simulink model "TST_AirCtl_Mon"  (R2016b)
settings: Solver=FixedStepDiscrete  StartTime=0.0  StopTime=simTime  FixedStep=sampleTime  RelTol=1e-3
values from neighbouring files (symbols this model uses):
  testCase = 1    [initTST_AirCtl_Mon_001.m]
libraries: simulink x8, UnitTest_Lib x6
settings Model: Creator=zhulinfeng  LastModifiedBy=zhulinfeng
settings DebuggingCC: SignalRangeChecking=error

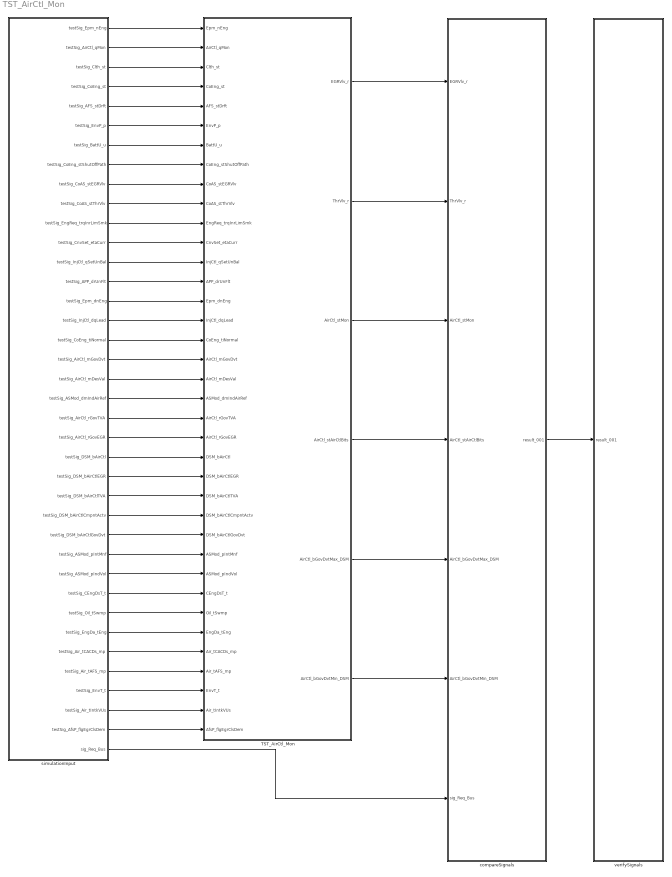
== system TST_AirCtl_Mon ==
  TST_AirCtl_Mon : Subsystem
  compareSignals : Subsystem
  simulationInput : Subsystem
  verifySignals : Subsystem
  wires:
  simulationInput/1(testSig_Epm_nEng) -> TST_AirCtl_Mon/1(Epm_nEng)
  simulationInput/2(testSig_AirCtl_qMon) -> TST_AirCtl_Mon/2(AirCtl_qMon)
  simulationInput/3(testSig_Clth_st) -> TST_AirCtl_Mon/3(Clth_st)
  simulationInput/4(testSig_CoEng_st) -> TST_AirCtl_Mon/4(CoEng_st)
  simulationInput/5(testSig_AFS_stDrft) -> TST_AirCtl_Mon/5(AFS_stDrft)
  simulationInput/6(testSig_EnvP_p) -> TST_AirCtl_Mon/6(EnvP_p)
  simulationInput/7(testSig_BattU_u) -> TST_AirCtl_Mon/7(BattU_u)
  simulationInput/8(testSig_CoEng_stShutOffPath) -> TST_AirCtl_Mon/8(CoEng_stShutOffPath)
  simulationInput/9(testSig_CoAS_stEGRVlv) -> TST_AirCtl_Mon/9(CoAS_stEGRVlv)
  simulationInput/10(testSig_CoAS_stThrVlv) -> TST_AirCtl_Mon/10(CoAS_stThrVlv)
  simulationInput/11(testSig_EngReq_trqInrLimSmk) -> TST_AirCtl_Mon/11(EngReq_trqInrLimSmk)
  simulationInput/12(testSig_CnvSet_etaCurr) -> TST_AirCtl_Mon/12(CnvSet_etaCurr)
  simulationInput/13(testSig_InjCtl_qSetUnBal) -> TST_AirCtl_Mon/13(InjCtl_qSetUnBal)
  simulationInput/14(testSig_APP_drUnFlt) -> TST_AirCtl_Mon/14(APP_drUnFlt)
  simulationInput/15(testSig_Epm_dnEng) -> TST_AirCtl_Mon/15(Epm_dnEng)
  simulationInput/16(testSig_InjCtl_dqLead) -> TST_AirCtl_Mon/16(InjCtl_dqLead)
  simulationInput/17(testSig_CoEng_tiNormal) -> TST_AirCtl_Mon/17(CoEng_tiNormal)
  simulationInput/18(testSig_AirCtl_mGovDvt) -> TST_AirCtl_Mon/18(AirCtl_mGovDvt)
  simulationInput/19(testSig_AirCtl_mDesVal) -> TST_AirCtl_Mon/19(AirCtl_mDesVal)
  simulationInput/20(testSig_ASMod_dmIndAirRef) -> TST_AirCtl_Mon/20(ASMod_dmIndAirRef)
  simulationInput/21(testSig_AirCtl_rGovTVA) -> TST_AirCtl_Mon/21(AirCtl_rGovTVA)
  simulationInput/22(testSig_AirCtl_rGovEGR) -> TST_AirCtl_Mon/22(AirCtl_rGovEGR)
  simulationInput/23(testSig_DSM_bAirCtl) -> TST_AirCtl_Mon/23(DSM_bAirCtl)
  simulationInput/24(testSig_DSM_bAirCtlEGR) -> TST_AirCtl_Mon/24(DSM_bAirCtlEGR)
  simulationInput/25(testSig_DSM_bAirCtlTVA) -> TST_AirCtl_Mon/25(DSM_bAirCtlTVA)
  simulationInput/26(testSig_DSM_bAirCtlCmpntActv) -> TST_AirCtl_Mon/26(DSM_bAirCtlCmpntActv)
  simulationInput/27(testSig_DSM_bAirCtlGovDvt) -> TST_AirCtl_Mon/27(DSM_bAirCtlGovDvt)
  simulationInput/28(testSig_ASMod_pIntMnf) -> TST_AirCtl_Mon/28(ASMod_pIntMnf)
  simulationInput/29(testSig_ASMod_pIndVol) -> TST_AirCtl_Mon/29(ASMod_pIndVol)
  simulationInput/30(testSig_CEngDsT_t) -> TST_AirCtl_Mon/30(CEngDsT_t)
  simulationInput/31(testSig_Oil_tSwmp) -> TST_AirCtl_Mon/31(Oil_tSwmp)
  simulationInput/32(testSig_EngDa_tEng) -> TST_AirCtl_Mon/32(EngDa_tEng)
  simulationInput/33(testSig_Air_tCACDs_mp) -> TST_AirCtl_Mon/33(Air_tCACDs_mp)
  simulationInput/34(testSig_Air_tAFS_mp) -> TST_AirCtl_Mon/34(Air_tAFS_mp)
  simulationInput/35(testSig_EnvT_t) -> TST_AirCtl_Mon/35(EnvT_t)
  simulationInput/36(testSig_Air_tIntkVUs) -> TST_AirCtl_Mon/36(Air_tIntkVUs)
  simulationInput/37(testSig_AfsP_flgEgrClsDem) -> TST_AirCtl_Mon/37(AfsP_flgEgrClsDem)
  TST_AirCtl_Mon/1(EGRVlv_r) -> compareSignals/1(EGRVlv_r)
  TST_AirCtl_Mon/2(ThrVlv_r) -> compareSignals/2(ThrVlv_r)
  TST_AirCtl_Mon/3(AirCtl_stMon) -> compareSignals/3(AirCtl_stMon)
  TST_AirCtl_Mon/4(AirCtl_stAirCtlBits) -> compareSignals/4(AirCtl_stAirCtlBits)
  TST_AirCtl_Mon/5(AirCtl_bGovDvtMax_DSM) -> compareSignals/5(AirCtl_bGovDvtMax_DSM)
  TST_AirCtl_Mon/6(AirCtl_bGovDvtMin_DSM) -> compareSignals/6(AirCtl_bGovDvtMin_DSM)
  simulationInput/38(sig_Req_Bus) -> compareSignals/7(sig_Req_Bus)
  compareSignals/1(result_001) -> verifySignals/1(result_001)

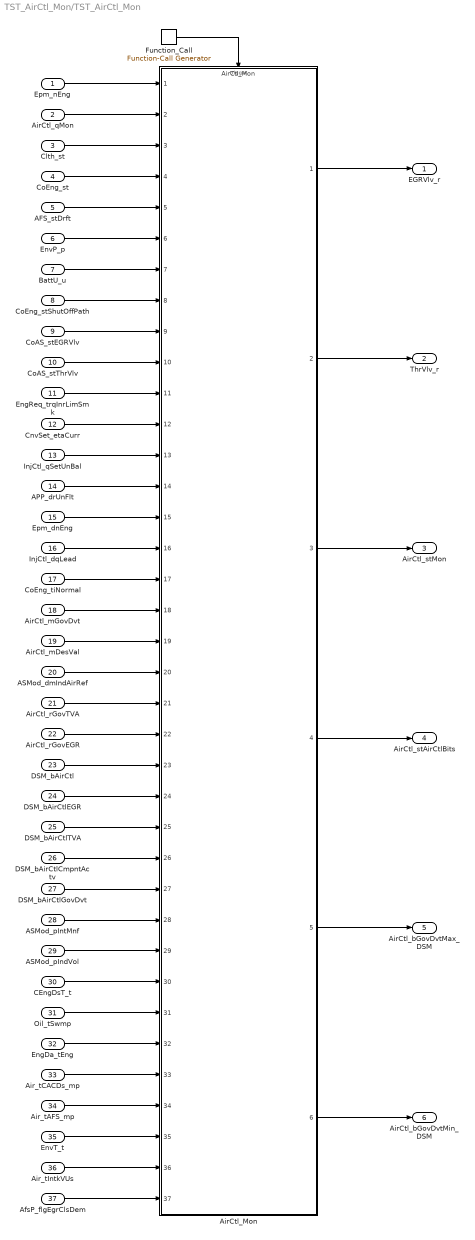
== system TST_AirCtl_Mon/TST_AirCtl_Mon ==
  Epm_nEng : Inport
  AirCtl_qMon : Inport  Port=2
  Clth_st : Inport  Port=3
  CoEng_st : Inport  Port=4
  AFS_stDrft : Inport  Port=5
  EnvP_p : Inport  Port=6
  BattU_u : Inport  Port=7
  CoEng_stShutOffPath : Inport  Port=8
  CoAS_stEGRVlv : Inport  Port=9
  CoAS_stThrVlv : Inport  Port=10
  EngReq_trqInrLimSmk : Inport  Port=11
  CnvSet_etaCurr : Inport  Port=12
  InjCtl_qSetUnBal : Inport  Port=13
  APP_drUnFlt : Inport  Port=14
  Epm_dnEng : Inport  Port=15
  InjCtl_dqLead : Inport  Port=16
  CoEng_tiNormal : Inport  Port=17
  AirCtl_mGovDvt : Inport  Port=18
  AirCtl_mDesVal : Inport  Port=19
  ASMod_dmIndAirRef : Inport  Port=20
  AirCtl_rGovTVA : Inport  Port=21
  AirCtl_rGovEGR : Inport  Port=22
  DSM_bAirCtl : Inport  Port=23
  DSM_bAirCtlEGR : Inport  Port=24
  DSM_bAirCtlTVA : Inport  Port=25
  DSM_bAirCtlCmpntActv : Inport  Port=26
  DSM_bAirCtlGovDvt : Inport  Port=27
  ASMod_pIntMnf : Inport  Port=28
  ASMod_pIndVol : Inport  Port=29
  CEngDsT_t : Inport  Port=30
  Oil_tSwmp : Inport  Port=31
  EngDa_tEng : Inport  Port=32
  Air_tCACDs_mp : Inport  Port=33
  Air_tAFS_mp : Inport  Port=34
  EnvT_t : Inport  Port=35
  Air_tIntkVUs : Inport  Port=36
  AfsP_flgEgrClsDem : Inport  Port=37
  AirCtl_Mon : ModelReference  ModelNameDialog=AirCtl_Mon  SimulationMode=Normal  ModelReferenceVersion=1.83  TriggerPortName=function  TriggerPortTriggerType=function-call  TriggerPortStatesWhenEnabling=held
  Function_Call : simulink/Ports & Subsystems/Function-Call Generator  sample_time=sampleTime  numberOfIterations=1
  EGRVlv_r : Outport
  ThrVlv_r : Outport  Port=2
  AirCtl_stMon : Outport  Port=3
  AirCtl_stAirCtlBits : Outport  Port=4
  AirCtl_bGovDvtMax_DSM : Outport  Port=5
  AirCtl_bGovDvtMin_DSM : Outport  Port=6
  wires:
  Function_Call/1 -> AirCtl_Mon/Trigger
  Epm_nEng/1 -> AirCtl_Mon/1
  AirCtl_qMon/1 -> AirCtl_Mon/2
  Clth_st/1 -> AirCtl_Mon/3
  CoEng_st/1 -> AirCtl_Mon/4
  AFS_stDrft/1 -> AirCtl_Mon/5
  EnvP_p/1 -> AirCtl_Mon/6
  BattU_u/1 -> AirCtl_Mon/7
  CoEng_stShutOffPath/1 -> AirCtl_Mon/8
  CoAS_stEGRVlv/1 -> AirCtl_Mon/9
  CoAS_stThrVlv/1 -> AirCtl_Mon/10
  EngReq_trqInrLimSmk/1 -> AirCtl_Mon/11
  CnvSet_etaCurr/1 -> AirCtl_Mon/12
  InjCtl_qSetUnBal/1 -> AirCtl_Mon/13
  APP_drUnFlt/1 -> AirCtl_Mon/14
  Epm_dnEng/1 -> AirCtl_Mon/15
  InjCtl_dqLead/1 -> AirCtl_Mon/16
  CoEng_tiNormal/1 -> AirCtl_Mon/17
  AirCtl_mGovDvt/1 -> AirCtl_Mon/18
  AirCtl_mDesVal/1 -> AirCtl_Mon/19
  ASMod_dmIndAirRef/1 -> AirCtl_Mon/20
  AirCtl_rGovTVA/1 -> AirCtl_Mon/21
  AirCtl_rGovEGR/1 -> AirCtl_Mon/22
  DSM_bAirCtl/1 -> AirCtl_Mon/23
  DSM_bAirCtlEGR/1 -> AirCtl_Mon/24
  DSM_bAirCtlTVA/1 -> AirCtl_Mon/25
  DSM_bAirCtlCmpntActv/1 -> AirCtl_Mon/26
  DSM_bAirCtlGovDvt/1 -> AirCtl_Mon/27
  ASMod_pIntMnf/1 -> AirCtl_Mon/28
  ASMod_pIndVol/1 -> AirCtl_Mon/29
  CEngDsT_t/1 -> AirCtl_Mon/30
  Oil_tSwmp/1 -> AirCtl_Mon/31
  EngDa_tEng/1 -> AirCtl_Mon/32
  Air_tCACDs_mp/1 -> AirCtl_Mon/33
  Air_tAFS_mp/1 -> AirCtl_Mon/34
  EnvT_t/1 -> AirCtl_Mon/35
  Air_tIntkVUs/1 -> AirCtl_Mon/36
  AfsP_flgEgrClsDem/1 -> AirCtl_Mon/37
  AirCtl_Mon/1 -> EGRVlv_r/1
  AirCtl_Mon/2 -> ThrVlv_r/1
  AirCtl_Mon/3 -> AirCtl_stMon/1
  AirCtl_Mon/4 -> AirCtl_stAirCtlBits/1
  AirCtl_Mon/5 -> AirCtl_bGovDvtMax_DSM/1
  AirCtl_Mon/6 -> AirCtl_bGovDvtMin_DSM/1

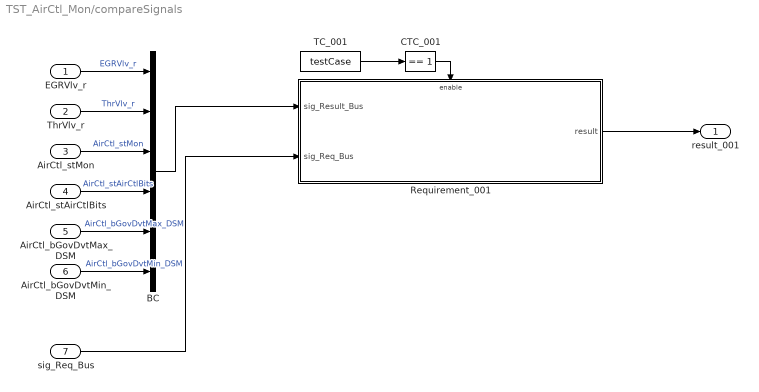
== system TST_AirCtl_Mon/compareSignals ==
  EGRVlv_r : Inport
  ThrVlv_r : Inport  Port=2
  AirCtl_stMon : Inport  Port=3
  AirCtl_stAirCtlBits : Inport  Port=4
  AirCtl_bGovDvtMax_DSM : Inport  Port=5
  AirCtl_bGovDvtMin_DSM : Inport  Port=6
  sig_Req_Bus : Inport  Port=7
  BC : BusCreator  Inputs=6
  CTC_001 : simulink/Logic and Bit Operations/Compare To Constant  relop===  const=1  OutDataTypeStr=boolean
  Requirement_001 : Subsystem
  TC_001 : Constant  Value=testCase
  result_001 : Outport
  wires:
  EGRVlv_r/1 -> BC/1  "EGRVlv_r"
  ThrVlv_r/1 -> BC/2  "ThrVlv_r"
  AirCtl_stMon/1 -> BC/3  "AirCtl_stMon"
  AirCtl_stAirCtlBits/1 -> BC/4  "AirCtl_stAirCtlBits"
  AirCtl_bGovDvtMax_DSM/1 -> BC/5  "AirCtl_bGovDvtMax_DSM"
  AirCtl_bGovDvtMin_DSM/1 -> BC/6  "AirCtl_bGovDvtMin_DSM"
  TC_001/1 -> CTC_001/1
  CTC_001/1 -> Requirement_001/Enable
  sig_Req_Bus/1 -> Requirement_001/2(sig_Req_Bus)
  BC/1 -> Requirement_001/1(sig_Result_Bus)
  Requirement_001/1(result) -> result_001/1

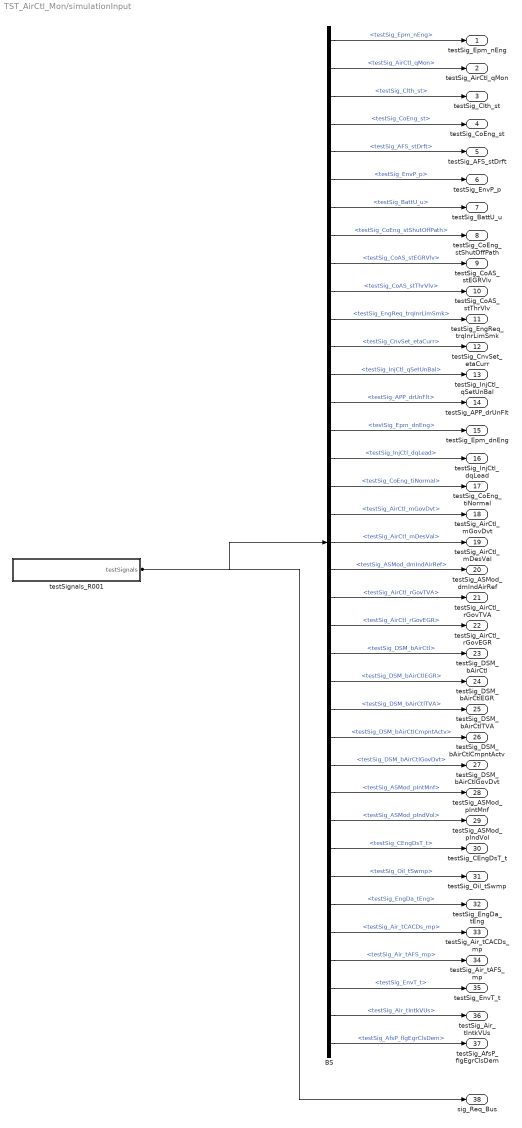
== system TST_AirCtl_Mon/simulationInput ==
  BS : BusSelector  OutputSignals=testSig_Epm_nEng,testSig_AirCtl_qMon,testSig_Clth_st,testSig_CoEng_st,testSig_AFS_stDrft,testSig_EnvP_p,testSig_BattU_u,testSig_CoEng_stShutOffPath,testSig_CoAS_stEGRVlv,testSig_CoAS_stThrVlv,testSig_EngReq_trqInrLimSmk,testSig_CnvSet_etaCurr,testSig_InjCtl_qSetUnBal,testSig_APP_drUnFlt,testSig_Epm_dnEng,testSig_InjCtl_dqLead,testSig_CoEng_tiNormal,testSig_AirCtl_mGovDvt,testSig_AirCtl_mDesVal,testSig_ASMod_dmIndAirRef,testSig_AirCtl_rGovTVA,testSig_AirCtl_rGovEGR,testSig_DSM_bAirCtl,testSig_DSM_bAirCtlEGR,testSig_DSM_bAirCtlTVA,testSig_DSM_bAirCtlCmpntActv,testSig_DSM_bAirCtlGovDvt,testSig_ASMod_pIntMnf,testSig_ASMod_pIndVol,testSig_CEngDsT_t,testSig_Oil_tSwmp,testSig_EngDa_tEng,testSig_Air_tCACDs_mp,testSig_Air_tAFS_mp,testSig_EnvT_t,testSig_Air_tIntkVUs,testSig_AfsP_flgEgrClsDem
  testSignals_R001 : Subsystem
  testSig_Epm_nEng : Outport
  testSig_AirCtl_qMon : Outport  Port=2
  testSig_Clth_st : Outport  Port=3
  testSig_CoEng_st : Outport  Port=4
  testSig_AFS_stDrft : Outport  Port=5
  testSig_EnvP_p : Outport  Port=6
  testSig_BattU_u : Outport  Port=7
  testSig_CoEng_stShutOffPath : Outport  Port=8
  testSig_CoAS_stEGRVlv : Outport  Port=9
  testSig_CoAS_stThrVlv : Outport  Port=10
  testSig_EngReq_trqInrLimSmk : Outport  Port=11
  testSig_CnvSet_etaCurr : Outport  Port=12
  testSig_InjCtl_qSetUnBal : Outport  Port=13
  testSig_APP_drUnFlt : Outport  Port=14
  testSig_Epm_dnEng : Outport  Port=15
  testSig_InjCtl_dqLead : Outport  Port=16
  testSig_CoEng_tiNormal : Outport  Port=17
  testSig_AirCtl_mGovDvt : Outport  Port=18
  testSig_AirCtl_mDesVal : Outport  Port=19
  testSig_ASMod_dmIndAirRef : Outport  Port=20
  testSig_AirCtl_rGovTVA : Outport  Port=21
  testSig_AirCtl_rGovEGR : Outport  Port=22
  testSig_DSM_bAirCtl : Outport  Port=23
  testSig_DSM_bAirCtlEGR : Outport  Port=24
  testSig_DSM_bAirCtlTVA : Outport  Port=25
  testSig_DSM_bAirCtlCmpntActv : Outport  Port=26
  testSig_DSM_bAirCtlGovDvt : Outport  Port=27
  testSig_ASMod_pIntMnf : Outport  Port=28
  testSig_ASMod_pIndVol : Outport  Port=29
  testSig_CEngDsT_t : Outport  Port=30
  testSig_Oil_tSwmp : Outport  Port=31
  testSig_EngDa_tEng : Outport  Port=32
  testSig_Air_tCACDs_mp : Outport  Port=33
  testSig_Air_tAFS_mp : Outport  Port=34
  testSig_EnvT_t : Outport  Port=35
  testSig_Air_tIntkVUs : Outport  Port=36
  testSig_AfsP_flgEgrClsDem : Outport  Port=37
  sig_Req_Bus : Outport  Port=38
  wires:
  BS/1 -> testSig_Epm_nEng/1  "<testSig_Epm_nEng>"
  BS/2 -> testSig_AirCtl_qMon/1  "<testSig_AirCtl_qMon>"
  BS/3 -> testSig_Clth_st/1  "<testSig_Clth_st>"
  BS/4 -> testSig_CoEng_st/1  "<testSig_CoEng_st>"
  BS/5 -> testSig_AFS_stDrft/1  "<testSig_AFS_stDrft>"
  BS/6 -> testSig_EnvP_p/1  "<testSig_EnvP_p>"
  BS/7 -> testSig_BattU_u/1  "<testSig_BattU_u>"
  BS/8 -> testSig_CoEng_stShutOffPath/1  "<testSig_CoEng_stShutOffPath>"
  BS/9 -> testSig_CoAS_stEGRVlv/1  "<testSig_CoAS_stEGRVlv>"
  BS/10 -> testSig_CoAS_stThrVlv/1  "<testSig_CoAS_stThrVlv>"
  BS/11 -> testSig_EngReq_trqInrLimSmk/1  "<testSig_EngReq_trqInrLimSmk>"
  BS/12 -> testSig_CnvSet_etaCurr/1  "<testSig_CnvSet_etaCurr>"
  BS/13 -> testSig_InjCtl_qSetUnBal/1  "<testSig_InjCtl_qSetUnBal>"
  BS/14 -> testSig_APP_drUnFlt/1  "<testSig_APP_drUnFlt>"
  BS/15 -> testSig_Epm_dnEng/1  "<testSig_Epm_dnEng>"
  BS/16 -> testSig_InjCtl_dqLead/1  "<testSig_InjCtl_dqLead>"
  BS/17 -> testSig_CoEng_tiNormal/1  "<testSig_CoEng_tiNormal>"
  BS/18 -> testSig_AirCtl_mGovDvt/1  "<testSig_AirCtl_mGovDvt>"
  BS/19 -> testSig_AirCtl_mDesVal/1  "<testSig_AirCtl_mDesVal>"
  BS/20 -> testSig_ASMod_dmIndAirRef/1  "<testSig_ASMod_dmIndAirRef>"
  BS/21 -> testSig_AirCtl_rGovTVA/1  "<testSig_AirCtl_rGovTVA>"
  BS/22 -> testSig_AirCtl_rGovEGR/1  "<testSig_AirCtl_rGovEGR>"
  BS/23 -> testSig_DSM_bAirCtl/1  "<testSig_DSM_bAirCtl>"
  BS/24 -> testSig_DSM_bAirCtlEGR/1  "<testSig_DSM_bAirCtlEGR>"
  BS/25 -> testSig_DSM_bAirCtlTVA/1  "<testSig_DSM_bAirCtlTVA>"
  BS/26 -> testSig_DSM_bAirCtlCmpntActv/1  "<testSig_DSM_bAirCtlCmpntActv>"
  BS/27 -> testSig_DSM_bAirCtlGovDvt/1  "<testSig_DSM_bAirCtlGovDvt>"
  BS/28 -> testSig_ASMod_pIntMnf/1  "<testSig_ASMod_pIntMnf>"
  BS/29 -> testSig_ASMod_pIndVol/1  "<testSig_ASMod_pIndVol>"
  BS/30 -> testSig_CEngDsT_t/1  "<testSig_CEngDsT_t>"
  BS/31 -> testSig_Oil_tSwmp/1  "<testSig_Oil_tSwmp>"
  BS/32 -> testSig_EngDa_tEng/1  "<testSig_EngDa_tEng>"
  BS/33 -> testSig_Air_tCACDs_mp/1  "<testSig_Air_tCACDs_mp>"
  BS/34 -> testSig_Air_tAFS_mp/1  "<testSig_Air_tAFS_mp>"
  BS/35 -> testSig_EnvT_t/1  "<testSig_EnvT_t>"
  BS/36 -> testSig_Air_tIntkVUs/1  "<testSig_Air_tIntkVUs>"
  BS/37 -> testSig_AfsP_flgEgrClsDem/1  "<testSig_AfsP_flgEgrClsDem>"
  testSignals_R001/1(testSignals) -> BS/1, sig_Req_Bus/1

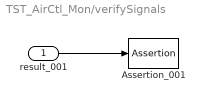
== system TST_AirCtl_Mon/verifySignals ==
  result_001 : Inport
  Assertion_001 : Assertion  Enabled=off
  wires:
  result_001/1 -> Assertion_001/1

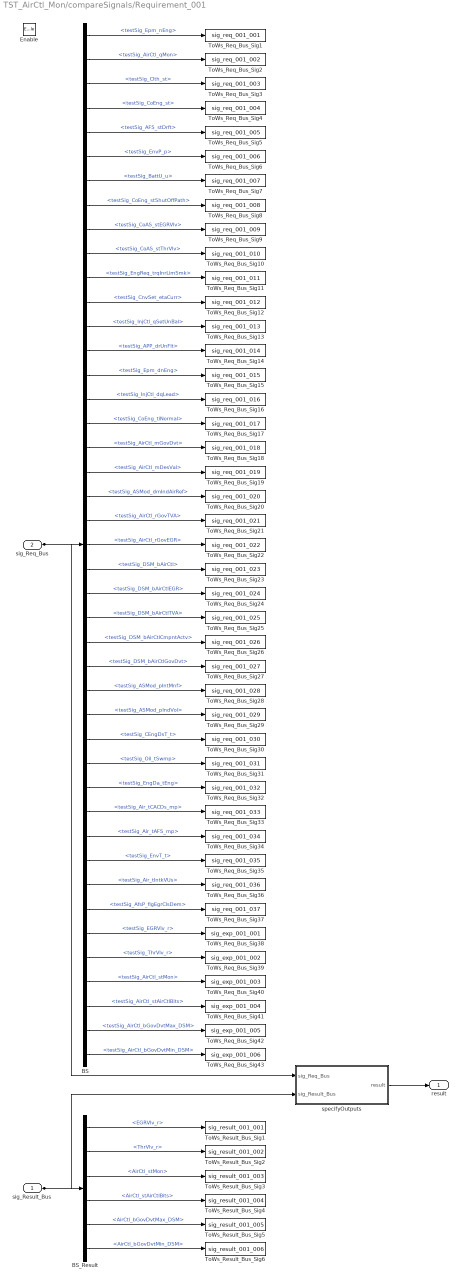
== system TST_AirCtl_Mon/compareSignals/Requirement_001 ==
  sig_Result_Bus : Inport
  sig_Req_Bus : Inport  Port=2
  Enable : EnablePort
  BS : BusSelector  OutputSignals=testSig_Epm_nEng,testSig_AirCtl_qMon,testSig_Clth_st,testSig_CoEng_st,testSig_AFS_stDrft,testSig_EnvP_p,testSig_BattU_u,testSig_CoEng_stShutOffPath,testSig_CoAS_stEGRVlv,testSig_CoAS_stThrVlv,testSig_EngReq_trqInrLimSmk,testSig_CnvSet_etaCurr,testSig_InjCtl_qSetUnBal,testSig_APP_drUnFlt,testSig_Epm_dnEng,testSig_InjCtl_dqLead,testSig_CoEng_tiNormal,testSig_AirCtl_mGovDvt,testSig_AirCtl_mDesVal,testSig_ASMod_dmIndAirRef,testSig_AirCtl_rGovTVA,testSig_AirCtl_rGovEGR,testSig_DSM_bAirCtl,testSig_DSM_bAirCtlEGR,testSig_DSM_bAirCtlTVA,testSig_DSM_bAirCtlCmpntActv,testSig_DSM_bAirCtlGovDvt,testSig_ASMod_pIntMnf,testSig_ASMod_pIndVol,testSig_CEngDsT_t,testSig_Oil_tSwmp,testSig_EngDa_tEng,testSig_Air_tCACDs_mp,testSig_Air_tAFS_mp,testSig_EnvT_t,testSig_Air_tIntkVUs,testSig_AfsP_flgEgrClsDem,testSig_EGRVlv_r,testSig_ThrVlv_r,testSig_AirCtl_stMon,testSig_AirCtl_stAirCtlBits,testSig_AirCtl_bGovDvtMax_DSM,testSig_AirCtl_bGovDvtMin_DSM
  BS_Result : BusSelector  OutputSignals=EGRVlv_r,ThrVlv_r,AirCtl_stMon,AirCtl_stAirCtlBits,AirCtl_bGovDvtMax_DSM,AirCtl_bGovDvtMin_DSM
  ToWs_Req_Bus_Sig1 : ToWorkspace  VariableName=sig_req_001_001  SaveFormat=Structure With Time
  ToWs_Req_Bus_Sig10 : ToWorkspace  VariableName=sig_req_001_010  SaveFormat=Structure With Time
  ToWs_Req_Bus_Sig11 : ToWorkspace  VariableName=sig_req_001_011  SaveFormat=Structure With Time
  ToWs_Req_Bus_Sig12 : ToWorkspace  VariableName=sig_req_001_012  SaveFormat=Structure With Time
  ToWs_Req_Bus_Sig13 : ToWorkspace  VariableName=sig_req_001_013  SaveFormat=Structure With Time
  ToWs_Req_Bus_Sig14 : ToWorkspace  VariableName=sig_req_001_014  SaveFormat=Structure With Time
  ToWs_Req_Bus_Sig15 : ToWorkspace  VariableName=sig_req_001_015  SaveFormat=Structure With Time
  ToWs_Req_Bus_Sig16 : ToWorkspace  VariableName=sig_req_001_016  SaveFormat=Structure With Time
  ToWs_Req_Bus_Sig17 : ToWorkspace  VariableName=sig_req_001_017  SaveFormat=Structure With Time
  ToWs_Req_Bus_Sig18 : ToWorkspace  VariableName=sig_req_001_018  SaveFormat=Structure With Time
  ToWs_Req_Bus_Sig19 : ToWorkspace  VariableName=sig_req_001_019  SaveFormat=Structure With Time
  ToWs_Req_Bus_Sig2 : ToWorkspace  VariableName=sig_req_001_002  SaveFormat=Structure With Time
  ToWs_Req_Bus_Sig20 : ToWorkspace  VariableName=sig_req_001_020  SaveFormat=Structure With Time
  ToWs_Req_Bus_Sig21 : ToWorkspace  VariableName=sig_req_001_021  SaveFormat=Structure With Time
  ToWs_Req_Bus_Sig22 : ToWorkspace  VariableName=sig_req_001_022  SaveFormat=Structure With Time
  ToWs_Req_Bus_Sig23 : ToWorkspace  VariableName=sig_req_001_023  SaveFormat=Structure With Time
  ToWs_Req_Bus_Sig24 : ToWorkspace  VariableName=sig_req_001_024  SaveFormat=Structure With Time
  ToWs_Req_Bus_Sig25 : ToWorkspace  VariableName=sig_req_001_025  SaveFormat=Structure With Time
  ToWs_Req_Bus_Sig26 : ToWorkspace  VariableName=sig_req_001_026  SaveFormat=Structure With Time
  ToWs_Req_Bus_Sig27 : ToWorkspace  VariableName=sig_req_001_027  SaveFormat=Structure With Time
  ToWs_Req_Bus_Sig28 : ToWorkspace  VariableName=sig_req_001_028  SaveFormat=Structure With Time
  ToWs_Req_Bus_Sig29 : ToWorkspace  VariableName=sig_req_001_029  SaveFormat=Structure With Time
  ToWs_Req_Bus_Sig3 : ToWorkspace  VariableName=sig_req_001_003  SaveFormat=Structure With Time
  ToWs_Req_Bus_Sig30 : ToWorkspace  VariableName=sig_req_001_030  SaveFormat=Structure With Time
  ToWs_Req_Bus_Sig31 : ToWorkspace  VariableName=sig_req_001_031  SaveFormat=Structure With Time
  ToWs_Req_Bus_Sig32 : ToWorkspace  VariableName=sig_req_001_032  SaveFormat=Structure With Time
  ToWs_Req_Bus_Sig33 : ToWorkspace  VariableName=sig_req_001_033  SaveFormat=Structure With Time
  ToWs_Req_Bus_Sig34 : ToWorkspace  VariableName=sig_req_001_034  SaveFormat=Structure With Time
  ToWs_Req_Bus_Sig35 : ToWorkspace  VariableName=sig_req_001_035  SaveFormat=Structure With Time
  ToWs_Req_Bus_Sig36 : ToWorkspace  VariableName=sig_req_001_036  SaveFormat=Structure With Time
  ToWs_Req_Bus_Sig37 : ToWorkspace  VariableName=sig_req_001_037  SaveFormat=Structure With Time
  ToWs_Req_Bus_Sig38 : ToWorkspace  VariableName=sig_exp_001_001  SaveFormat=Structure With Time
  ToWs_Req_Bus_Sig39 : ToWorkspace  VariableName=sig_exp_001_002  SaveFormat=Structure With Time
  ToWs_Req_Bus_Sig4 : ToWorkspace  VariableName=sig_req_001_004  SaveFormat=Structure With Time
  ToWs_Req_Bus_Sig40 : ToWorkspace  VariableName=sig_exp_001_003  SaveFormat=Structure With Time
  ToWs_Req_Bus_Sig41 : ToWorkspace  VariableName=sig_exp_001_004  SaveFormat=Structure With Time
  ToWs_Req_Bus_Sig42 : ToWorkspace  VariableName=sig_exp_001_005  SaveFormat=Structure With Time
  ToWs_Req_Bus_Sig43 : ToWorkspace  VariableName=sig_exp_001_006  SaveFormat=Structure With Time
  ToWs_Req_Bus_Sig5 : ToWorkspace  VariableName=sig_req_001_005  SaveFormat=Structure With Time
  ToWs_Req_Bus_Sig6 : ToWorkspace  VariableName=sig_req_001_006  SaveFormat=Structure With Time
  ToWs_Req_Bus_Sig7 : ToWorkspace  VariableName=sig_req_001_007  SaveFormat=Structure With Time
  ToWs_Req_Bus_Sig8 : ToWorkspace  VariableName=sig_req_001_008  SaveFormat=Structure With Time
  ToWs_Req_Bus_Sig9 : ToWorkspace  VariableName=sig_req_001_009  SaveFormat=Structure With Time
  ToWs_Result_Bus_Sig1 : ToWorkspace  VariableName=sig_result_001_001  SaveFormat=Structure With Time
  ToWs_Result_Bus_Sig2 : ToWorkspace  VariableName=sig_result_001_002  SaveFormat=Structure With Time
  ToWs_Result_Bus_Sig3 : ToWorkspace  VariableName=sig_result_001_003  SaveFormat=Structure With Time
  ToWs_Result_Bus_Sig4 : ToWorkspace  VariableName=sig_result_001_004  SaveFormat=Structure With Time
  ToWs_Result_Bus_Sig5 : ToWorkspace  VariableName=sig_result_001_005  SaveFormat=Structure With Time
  ToWs_Result_Bus_Sig6 : ToWorkspace  VariableName=sig_result_001_006  SaveFormat=Structure With Time
  specifyOutputs : Subsystem
  result : Outport
  wires:
  sig_Req_Bus/1 -> BS/1, specifyOutputs/1(sig_Req_Bus)
  BS/1 -> ToWs_Req_Bus_Sig1/1  "<testSig_Epm_nEng>"
  BS/2 -> ToWs_Req_Bus_Sig2/1  "<testSig_AirCtl_qMon>"
  BS/3 -> ToWs_Req_Bus_Sig3/1  "<testSig_Clth_st>"
  BS/4 -> ToWs_Req_Bus_Sig4/1  "<testSig_CoEng_st>"
  BS/5 -> ToWs_Req_Bus_Sig5/1  "<testSig_AFS_stDrft>"
  BS/6 -> ToWs_Req_Bus_Sig6/1  "<testSig_EnvP_p>"
  BS/7 -> ToWs_Req_Bus_Sig7/1  "<testSig_BattU_u>"
  BS/8 -> ToWs_Req_Bus_Sig8/1  "<testSig_CoEng_stShutOffPath>"
  BS/9 -> ToWs_Req_Bus_Sig9/1  "<testSig_CoAS_stEGRVlv>"
  BS/10 -> ToWs_Req_Bus_Sig10/1  "<testSig_CoAS_stThrVlv>"
  BS/11 -> ToWs_Req_Bus_Sig11/1  "<testSig_EngReq_trqInrLimSmk>"
  BS/12 -> ToWs_Req_Bus_Sig12/1  "<testSig_CnvSet_etaCurr>"
  BS/13 -> ToWs_Req_Bus_Sig13/1  "<testSig_InjCtl_qSetUnBal>"
  BS/14 -> ToWs_Req_Bus_Sig14/1  "<testSig_APP_drUnFlt>"
  BS/15 -> ToWs_Req_Bus_Sig15/1  "<testSig_Epm_dnEng>"
  BS/16 -> ToWs_Req_Bus_Sig16/1  "<testSig_InjCtl_dqLead>"
  BS/17 -> ToWs_Req_Bus_Sig17/1  "<testSig_CoEng_tiNormal>"
  BS/18 -> ToWs_Req_Bus_Sig18/1  "<testSig_AirCtl_mGovDvt>"
  BS/19 -> ToWs_Req_Bus_Sig19/1  "<testSig_AirCtl_mDesVal>"
  BS/20 -> ToWs_Req_Bus_Sig20/1  "<testSig_ASMod_dmIndAirRef>"
  BS/21 -> ToWs_Req_Bus_Sig21/1  "<testSig_AirCtl_rGovTVA>"
  BS/22 -> ToWs_Req_Bus_Sig22/1  "<testSig_AirCtl_rGovEGR>"
  BS/23 -> ToWs_Req_Bus_Sig23/1  "<testSig_DSM_bAirCtl>"
  BS/24 -> ToWs_Req_Bus_Sig24/1  "<testSig_DSM_bAirCtlEGR>"
  BS/25 -> ToWs_Req_Bus_Sig25/1  "<testSig_DSM_bAirCtlTVA>"
  BS/26 -> ToWs_Req_Bus_Sig26/1  "<testSig_DSM_bAirCtlCmpntActv>"
  BS/27 -> ToWs_Req_Bus_Sig27/1  "<testSig_DSM_bAirCtlGovDvt>"
  BS/28 -> ToWs_Req_Bus_Sig28/1  "<testSig_ASMod_pIntMnf>"
  BS/29 -> ToWs_Req_Bus_Sig29/1  "<testSig_ASMod_pIndVol>"
  BS/30 -> ToWs_Req_Bus_Sig30/1  "<testSig_CEngDsT_t>"
  BS/31 -> ToWs_Req_Bus_Sig31/1  "<testSig_Oil_tSwmp>"
  BS/32 -> ToWs_Req_Bus_Sig32/1  "<testSig_EngDa_tEng>"
  BS/33 -> ToWs_Req_Bus_Sig33/1  "<testSig_Air_tCACDs_mp>"
  BS/34 -> ToWs_Req_Bus_Sig34/1  "<testSig_Air_tAFS_mp>"
  BS/35 -> ToWs_Req_Bus_Sig35/1  "<testSig_EnvT_t>"
  BS/36 -> ToWs_Req_Bus_Sig36/1  "<testSig_Air_tIntkVUs>"
  BS/37 -> ToWs_Req_Bus_Sig37/1  "<testSig_AfsP_flgEgrClsDem>"
  BS/38 -> ToWs_Req_Bus_Sig38/1  "<testSig_EGRVlv_r>"
  BS/39 -> ToWs_Req_Bus_Sig39/1  "<testSig_ThrVlv_r>"
  BS/40 -> ToWs_Req_Bus_Sig40/1  "<testSig_AirCtl_stMon>"
  BS/41 -> ToWs_Req_Bus_Sig41/1  "<testSig_AirCtl_stAirCtlBits>"
  BS/42 -> ToWs_Req_Bus_Sig42/1  "<testSig_AirCtl_bGovDvtMax_DSM>"
  BS/43 -> ToWs_Req_Bus_Sig43/1  "<testSig_AirCtl_bGovDvtMin_DSM>"
  sig_Result_Bus/1 -> BS_Result/1, specifyOutputs/2(sig_Result_Bus)
  BS_Result/1 -> ToWs_Result_Bus_Sig1/1  "<EGRVlv_r>"
  BS_Result/2 -> ToWs_Result_Bus_Sig2/1  "<ThrVlv_r>"
  BS_Result/3 -> ToWs_Result_Bus_Sig3/1  "<AirCtl_stMon>"
  BS_Result/4 -> ToWs_Result_Bus_Sig4/1  "<AirCtl_stAirCtlBits>"
  BS_Result/5 -> ToWs_Result_Bus_Sig5/1  "<AirCtl_bGovDvtMax_DSM>"
  BS_Result/6 -> ToWs_Result_Bus_Sig6/1  "<AirCtl_bGovDvtMin_DSM>"
  specifyOutputs/1(result) -> result/1

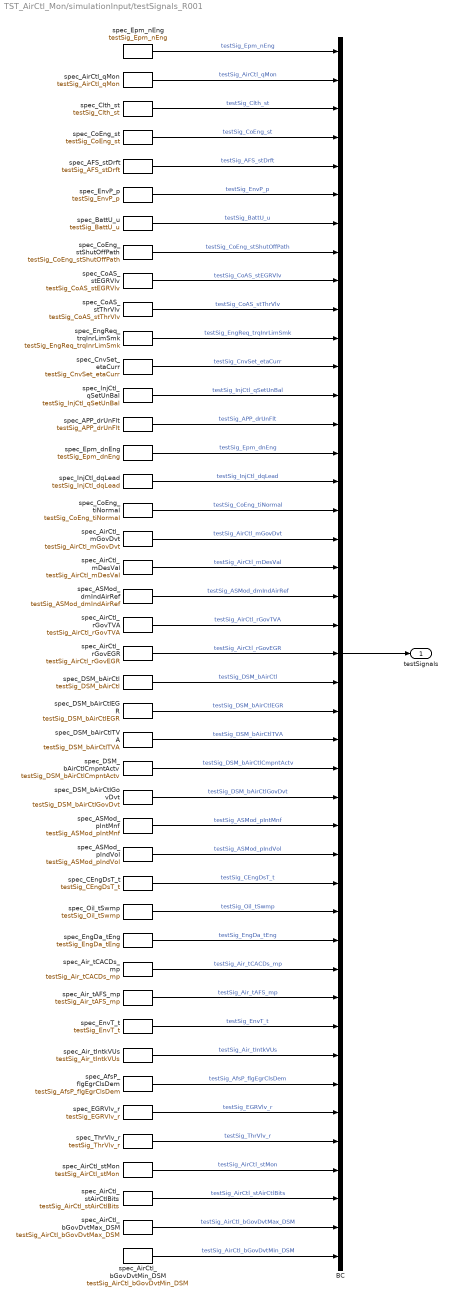
== system TST_AirCtl_Mon/simulationInput/testSignals_R001 ==
  BC : BusCreator  Inputs=43
  spec_AFS_stDrft : FromWorkspace  VariableName=testSig_AFS_stDrft  Interpolate=off  OutputAfterFinalValue=Holding final value
  spec_APP_drUnFlt : FromWorkspace  VariableName=testSig_APP_drUnFlt  Interpolate=off  OutputAfterFinalValue=Holding final value
  spec_ASMod_dmIndAirRef : FromWorkspace  VariableName=testSig_ASMod_dmIndAirRef  Interpolate=off  OutputAfterFinalValue=Holding final value
  spec_ASMod_pIndVol : FromWorkspace  VariableName=testSig_ASMod_pIndVol  Interpolate=off  OutputAfterFinalValue=Holding final value
  spec_ASMod_pIntMnf : FromWorkspace  VariableName=testSig_ASMod_pIntMnf  Interpolate=off  OutputAfterFinalValue=Holding final value
  spec_AfsP_flgEgrClsDem : FromWorkspace  VariableName=testSig_AfsP_flgEgrClsDem  Interpolate=off  OutputAfterFinalValue=Holding final value
  spec_AirCtl_bGovDvtMax_DSM : FromWorkspace  VariableName=testSig_AirCtl_bGovDvtMax_DSM  Interpolate=off  OutputAfterFinalValue=Holding final value
  spec_AirCtl_bGovDvtMin_DSM : FromWorkspace  VariableName=testSig_AirCtl_bGovDvtMin_DSM  Interpolate=off  OutputAfterFinalValue=Holding final value
  spec_AirCtl_mDesVal : FromWorkspace  VariableName=testSig_AirCtl_mDesVal  Interpolate=off  OutputAfterFinalValue=Holding final value
  spec_AirCtl_mGovDvt : FromWorkspace  VariableName=testSig_AirCtl_mGovDvt  Interpolate=off  OutputAfterFinalValue=Holding final value
  spec_AirCtl_qMon : FromWorkspace  VariableName=testSig_AirCtl_qMon  Interpolate=off  OutputAfterFinalValue=Holding final value
  spec_AirCtl_rGovEGR : FromWorkspace  VariableName=testSig_AirCtl_rGovEGR  Interpolate=off  OutputAfterFinalValue=Holding final value
  spec_AirCtl_rGovTVA : FromWorkspace  VariableName=testSig_AirCtl_rGovTVA  Interpolate=off  OutputAfterFinalValue=Holding final value
  spec_AirCtl_stAirCtlBits : FromWorkspace  VariableName=testSig_AirCtl_stAirCtlBits  Interpolate=off  OutputAfterFinalValue=Holding final value
  spec_AirCtl_stMon : FromWorkspace  VariableName=testSig_AirCtl_stMon  Interpolate=off  OutputAfterFinalValue=Holding final value
  spec_Air_tAFS_mp : FromWorkspace  VariableName=testSig_Air_tAFS_mp  Interpolate=off  OutputAfterFinalValue=Holding final value
  spec_Air_tCACDs_mp : FromWorkspace  VariableName=testSig_Air_tCACDs_mp  Interpolate=off  OutputAfterFinalValue=Holding final value
  spec_Air_tIntkVUs : FromWorkspace  VariableName=testSig_Air_tIntkVUs  Interpolate=off  OutputAfterFinalValue=Holding final value
  spec_BattU_u : FromWorkspace  VariableName=testSig_BattU_u  Interpolate=off  OutputAfterFinalValue=Holding final value
  spec_CEngDsT_t : FromWorkspace  VariableName=testSig_CEngDsT_t  Interpolate=off  OutputAfterFinalValue=Holding final value
  spec_Clth_st : FromWorkspace  VariableName=testSig_Clth_st  Interpolate=off  OutputAfterFinalValue=Holding final value
  spec_CnvSet_etaCurr : FromWorkspace  VariableName=testSig_CnvSet_etaCurr  Interpolate=off  OutputAfterFinalValue=Holding final value
  spec_CoAS_stEGRVlv : FromWorkspace  VariableName=testSig_CoAS_stEGRVlv  Interpolate=off  OutputAfterFinalValue=Holding final value
  spec_CoAS_stThrVlv : FromWorkspace  VariableName=testSig_CoAS_stThrVlv  Interpolate=off  OutputAfterFinalValue=Holding final value
  spec_CoEng_st : FromWorkspace  VariableName=testSig_CoEng_st  Interpolate=off  OutputAfterFinalValue=Holding final value
  spec_CoEng_stShutOffPath : FromWorkspace  VariableName=testSig_CoEng_stShutOffPath  Interpolate=off  OutputAfterFinalValue=Holding final value
  spec_CoEng_tiNormal : FromWorkspace  VariableName=testSig_CoEng_tiNormal  Interpolate=off  OutputAfterFinalValue=Holding final value
  spec_DSM_bAirCtl : FromWorkspace  VariableName=testSig_DSM_bAirCtl  Interpolate=off  OutputAfterFinalValue=Holding final value
  spec_DSM_bAirCtlCmpntActv : FromWorkspace  VariableName=testSig_DSM_bAirCtlCmpntActv  Interpolate=off  OutputAfterFinalValue=Holding final value
  spec_DSM_bAirCtlEGR : FromWorkspace  VariableName=testSig_DSM_bAirCtlEGR  Interpolate=off  OutputAfterFinalValue=Holding final value
  spec_DSM_bAirCtlGovDvt : FromWorkspace  VariableName=testSig_DSM_bAirCtlGovDvt  Interpolate=off  OutputAfterFinalValue=Holding final value
  spec_DSM_bAirCtlTVA : FromWorkspace  VariableName=testSig_DSM_bAirCtlTVA  Interpolate=off  OutputAfterFinalValue=Holding final value
  spec_EGRVlv_r : FromWorkspace  VariableName=testSig_EGRVlv_r  Interpolate=off  OutputAfterFinalValue=Holding final value
  spec_EngDa_tEng : FromWorkspace  VariableName=testSig_EngDa_tEng  Interpolate=off  OutputAfterFinalValue=Holding final value
  spec_EngReq_trqInrLimSmk : FromWorkspace  VariableName=testSig_EngReq_trqInrLimSmk  Interpolate=off  OutputAfterFinalValue=Holding final value
  spec_EnvP_p : FromWorkspace  VariableName=testSig_EnvP_p  Interpolate=off  OutputAfterFinalValue=Holding final value
  spec_EnvT_t : FromWorkspace  VariableName=testSig_EnvT_t  Interpolate=off  OutputAfterFinalValue=Holding final value
  spec_Epm_dnEng : FromWorkspace  VariableName=testSig_Epm_dnEng  Interpolate=off  OutputAfterFinalValue=Holding final value
  spec_Epm_nEng : FromWorkspace  VariableName=testSig_Epm_nEng  Interpolate=off  OutputAfterFinalValue=Holding final value
  spec_InjCtl_dqLead : FromWorkspace  VariableName=testSig_InjCtl_dqLead  Interpolate=off  OutputAfterFinalValue=Holding final value
  spec_InjCtl_qSetUnBal : FromWorkspace  VariableName=testSig_InjCtl_qSetUnBal  Interpolate=off  OutputAfterFinalValue=Holding final value
  spec_Oil_tSwmp : FromWorkspace  VariableName=testSig_Oil_tSwmp  Interpolate=off  OutputAfterFinalValue=Holding final value
  spec_ThrVlv_r : FromWorkspace  VariableName=testSig_ThrVlv_r  Interpolate=off  OutputAfterFinalValue=Holding final value
  testSignals : Outport
  wires:
  BC/1 -> testSignals/1
  spec_Epm_nEng/1 -> BC/1  "testSig_Epm_nEng"
  spec_AirCtl_qMon/1 -> BC/2  "testSig_AirCtl_qMon"
  spec_Clth_st/1 -> BC/3  "testSig_Clth_st"
  spec_CoEng_st/1 -> BC/4  "testSig_CoEng_st"
  spec_AFS_stDrft/1 -> BC/5  "testSig_AFS_stDrft"
  spec_EnvP_p/1 -> BC/6  "testSig_EnvP_p"
  spec_BattU_u/1 -> BC/7  "testSig_BattU_u"
  spec_CoEng_stShutOffPath/1 -> BC/8  "testSig_CoEng_stShutOffPath"
  spec_CoAS_stEGRVlv/1 -> BC/9  "testSig_CoAS_stEGRVlv"
  spec_CoAS_stThrVlv/1 -> BC/10  "testSig_CoAS_stThrVlv"
  spec_EngReq_trqInrLimSmk/1 -> BC/11  "testSig_EngReq_trqInrLimSmk"
  spec_CnvSet_etaCurr/1 -> BC/12  "testSig_CnvSet_etaCurr"
  spec_InjCtl_qSetUnBal/1 -> BC/13  "testSig_InjCtl_qSetUnBal"
  spec_APP_drUnFlt/1 -> BC/14  "testSig_APP_drUnFlt"
  spec_Epm_dnEng/1 -> BC/15  "testSig_Epm_dnEng"
  spec_InjCtl_dqLead/1 -> BC/16  "testSig_InjCtl_dqLead"
  spec_CoEng_tiNormal/1 -> BC/17  "testSig_CoEng_tiNormal"
  spec_AirCtl_mGovDvt/1 -> BC/18  "testSig_AirCtl_mGovDvt"
  spec_AirCtl_mDesVal/1 -> BC/19  "testSig_AirCtl_mDesVal"
  spec_ASMod_dmIndAirRef/1 -> BC/20  "testSig_ASMod_dmIndAirRef"
  spec_AirCtl_rGovTVA/1 -> BC/21  "testSig_AirCtl_rGovTVA"
  spec_AirCtl_rGovEGR/1 -> BC/22  "testSig_AirCtl_rGovEGR"
  spec_DSM_bAirCtl/1 -> BC/23  "testSig_DSM_bAirCtl"
  spec_DSM_bAirCtlEGR/1 -> BC/24  "testSig_DSM_bAirCtlEGR"
  spec_DSM_bAirCtlTVA/1 -> BC/25  "testSig_DSM_bAirCtlTVA"
  spec_DSM_bAirCtlCmpntActv/1 -> BC/26  "testSig_DSM_bAirCtlCmpntActv"
  spec_DSM_bAirCtlGovDvt/1 -> BC/27  "testSig_DSM_bAirCtlGovDvt"
  spec_ASMod_pIntMnf/1 -> BC/28  "testSig_ASMod_pIntMnf"
  spec_ASMod_pIndVol/1 -> BC/29  "testSig_ASMod_pIndVol"
  spec_CEngDsT_t/1 -> BC/30  "testSig_CEngDsT_t"
  spec_Oil_tSwmp/1 -> BC/31  "testSig_Oil_tSwmp"
  spec_EngDa_tEng/1 -> BC/32  "testSig_EngDa_tEng"
  spec_Air_tCACDs_mp/1 -> BC/33  "testSig_Air_tCACDs_mp"
  spec_Air_tAFS_mp/1 -> BC/34  "testSig_Air_tAFS_mp"
  spec_EnvT_t/1 -> BC/35  "testSig_EnvT_t"
  spec_Air_tIntkVUs/1 -> BC/36  "testSig_Air_tIntkVUs"
  spec_AfsP_flgEgrClsDem/1 -> BC/37  "testSig_AfsP_flgEgrClsDem"
  spec_EGRVlv_r/1 -> BC/38  "testSig_EGRVlv_r"
  spec_ThrVlv_r/1 -> BC/39  "testSig_ThrVlv_r"
  spec_AirCtl_stMon/1 -> BC/40  "testSig_AirCtl_stMon"
  spec_AirCtl_stAirCtlBits/1 -> BC/41  "testSig_AirCtl_stAirCtlBits"
  spec_AirCtl_bGovDvtMax_DSM/1 -> BC/42  "testSig_AirCtl_bGovDvtMax_DSM"
  spec_AirCtl_bGovDvtMin_DSM/1 -> BC/43  "testSig_AirCtl_bGovDvtMin_DSM"

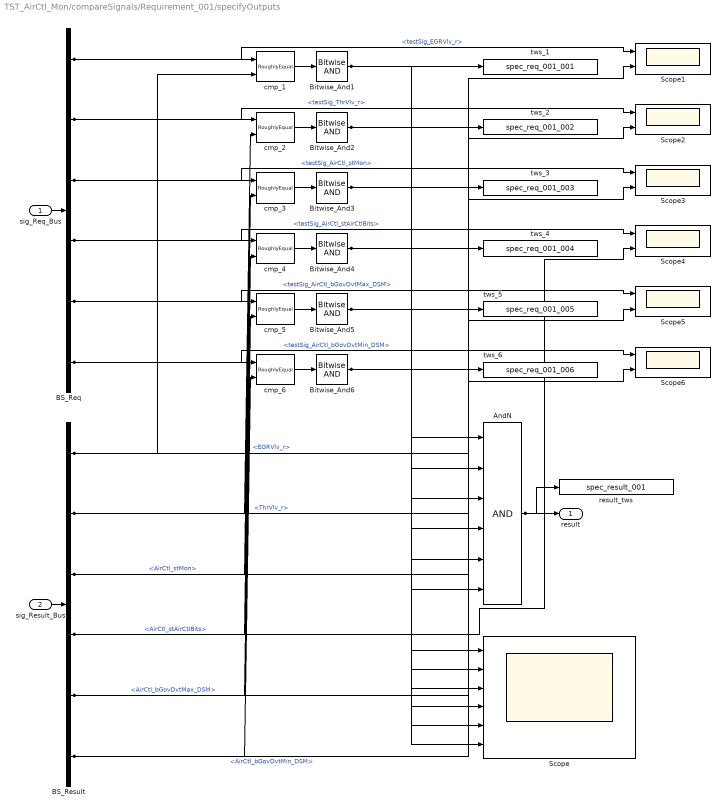
== system TST_AirCtl_Mon/compareSignals/Requirement_001/specifyOutputs ==
  sig_Req_Bus : Inport
  sig_Result_Bus : Inport  Port=2
  AndN : Logic  Inputs=6
  BS_Req : BusSelector  OutputSignals=testSig_EGRVlv_r,testSig_ThrVlv_r,testSig_AirCtl_stMon,testSig_AirCtl_stAirCtlBits,testSig_AirCtl_bGovDvtMax_DSM,testSig_AirCtl_bGovDvtMin_DSM
  BS_Result : BusSelector  OutputSignals=EGRVlv_r,ThrVlv_r,AirCtl_stMon,AirCtl_stAirCtlBits,AirCtl_bGovDvtMax_DSM,AirCtl_bGovDvtMin_DSM
  Bitwise_And{1..6} (6 alike) : simulink/Logic and Bit Operations/Bitwise Operator  logicop=AND  UseBitMask=off  BitMask=bin2dec('11011001')  BitMaskRealWorld=Stored Integer
  Scope : Scope  NumInputPorts=6
  Scope{1..6} (6 alike) : Scope  NumInputPorts=2
  cmp_{1..6} (6 alike) : UnitTest_Lib/RoughlyEqual  slope=0.1
  result_tws : ToWorkspace  VariableName=spec_result_001
  tws_1 : ToWorkspace  VariableName=spec_req_001_001
  tws_2 : ToWorkspace  VariableName=spec_req_001_002
  tws_3 : ToWorkspace  VariableName=spec_req_001_003
  tws_4 : ToWorkspace  VariableName=spec_req_001_004
  tws_5 : ToWorkspace  VariableName=spec_req_001_005
  tws_6 : ToWorkspace  VariableName=spec_req_001_006
  result : Outport
  wires:
  sig_Req_Bus/1 -> BS_Req/1
  sig_Result_Bus/1 -> BS_Result/1
  AndN/1 -> result/1, result_tws/1
  BS_Req/1 -> cmp_1/1, Scope1/1  "<testSig_EGRVlv_r>"
  BS_Result/1 -> cmp_1/2, Scope1/2  "<EGRVlv_r>"
  cmp_1/1 -> Bitwise_And1/1
  Bitwise_And1/1 -> tws_1/1, AndN/1, Scope/1
  BS_Req/2 -> cmp_2/1, Scope2/1  "<testSig_ThrVlv_r>"
  BS_Result/2 -> cmp_2/2, Scope2/2  "<ThrVlv_r>"
  cmp_2/1 -> Bitwise_And2/1
  Bitwise_And2/1 -> tws_2/1, AndN/2, Scope/2
  BS_Req/3 -> cmp_3/1, Scope3/1  "<testSig_AirCtl_stMon>"
  BS_Result/3 -> cmp_3/2, Scope3/2  "<AirCtl_stMon>"
  cmp_3/1 -> Bitwise_And3/1
  Bitwise_And3/1 -> tws_3/1, AndN/3, Scope/3
  BS_Req/4 -> cmp_4/1, Scope4/1  "<testSig_AirCtl_stAirCtlBits>"
  BS_Result/4 -> cmp_4/2, Scope4/2  "<AirCtl_stAirCtlBits>"
  cmp_4/1 -> Bitwise_And4/1
  Bitwise_And4/1 -> tws_4/1, AndN/4, Scope/4
  BS_Req/5 -> cmp_5/1, Scope5/1  "<testSig_AirCtl_bGovDvtMax_DSM>"
  BS_Result/5 -> cmp_5/2, Scope5/2  "<AirCtl_bGovDvtMax_DSM>"
  cmp_5/1 -> Bitwise_And5/1
  Bitwise_And5/1 -> tws_5/1, AndN/5, Scope/5
  BS_Req/6 -> cmp_6/1, Scope6/1  "<testSig_AirCtl_bGovDvtMin_DSM>"
  BS_Result/6 -> cmp_6/2, Scope6/2  "<AirCtl_bGovDvtMin_DSM>"
  cmp_6/1 -> Bitwise_And6/1
  Bitwise_And6/1 -> tws_6/1, AndN/6, Scope/6
